simulink model "gm_detector"  (R2022a)
settings: Solver=FixedStepDiscrete  StartTime=0.0  StopTime=simTime  RelTol=1e-3
model workspace (MAT data in the model file):
  Sig = Simulink.Signal
  Sig.DataType = 'auto'
  Sig.Dimensions = -1
  Sig.DimensionsMode = 'auto'
  Sig.Complexity = 'auto'
  Sig.SampleTime = -1
  Sig.SamplingMode = 'auto'
libraries: dspsrcs4 x2
settings Model: Creator=ASAHIN  LastModifiedBy=alpha
settings SolverCC: AlgebraicLoopSolver=TrustRegion
settings OptimizationCC: BlockReduction=off  ConditionallyExecuteInputs=off  DefaultParameterBehavior=Inlined  InheritOutputTypeSmallerThanSingle=on
settings DebuggingCC: AlgebraicLoopMsg=error  InheritedTsInSrcMsg=none  SingleTaskRateTransMsg=error  UnconnectedInputMsg=warning  UnconnectedOutputMsg=warning  UnconnectedLineMsg=warning  SFMachineParentedDataDiag=warning
settings HardwareCC: ProdBitPerPointer=32  ProdBitPerSizeT=32  ProdBitPerPtrDiffT=32  ProdLargestAtomicFloat=None  ProdIntDivRoundTo=Undefined  ProdEndianess=Unspecified  ProdWordSize=32  ProdHWDeviceType=ASIC/FPGA->ASIC/FPGA  TargetBitPerPointer=64  TargetBitPerSizeT=64  TargetBitPerPtrDiffT=64  TargetLongLongMode=on  TargetIntDivRoundTo=Zero  TargetEndianess=LittleEndian  TargetWordSize=64  TargetHWDeviceType=Custom Processor->MATLAB Host Computer  ProdEqTarget=off
settings RTWCC: DLArmComputeVersion=19.05

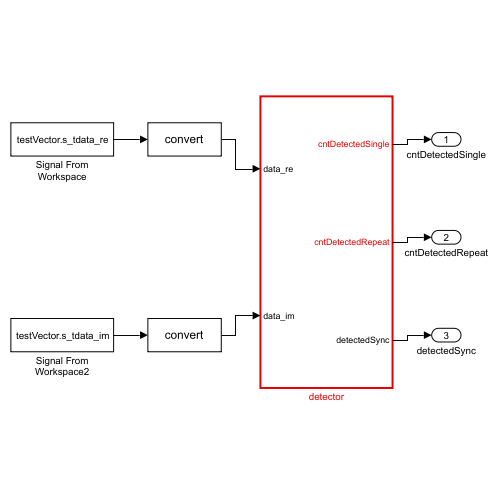
[thumbnail: Simulink's stored preview of the top-level diagram]
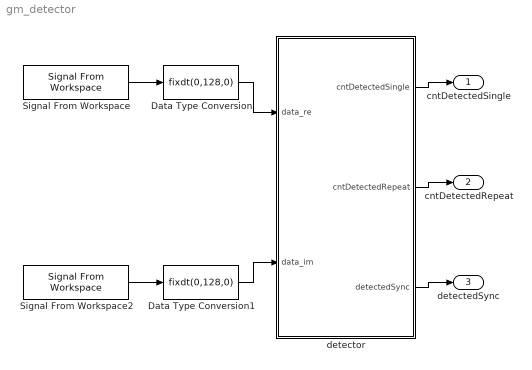
== system gm_detector ==
  Data Type Conversion : DataTypeConversion  OutDataTypeStr=fixdt(0,128,0)  SaturateOnIntegerOverflow=off  RndMeth=Floor
  Data Type Conversion1 : DataTypeConversion  OutDataTypeStr=fixdt(0,128,0)  SaturateOnIntegerOverflow=off  RndMeth=Floor
  Signal From Workspace : dspsrcs4/Signal From Workspace  X=testVector.s_tdata_re  Ts=1  nsamps=1  OutputAfterFinalValue=Setting to zero  ignoreOrWarnInputAndFrameLengths=off  OutputFrames=off
  Signal From Workspace2 : dspsrcs4/Signal From Workspace  X=testVector.s_tdata_im  Ts=1  nsamps=1  OutputAfterFinalValue=Setting to zero  ignoreOrWarnInputAndFrameLengths=off  OutputFrames=off
  detector : Subsystem  TreatAsAtomicUnit=on
  cntDetectedSingle : Outport
  cntDetectedRepeat : Outport  Port=2
  detectedSync : Outport  Port=3
  wires:
  Signal From Workspace/1 -> Data Type Conversion/1
  detector/1(cntDetectedSingle) -> cntDetectedSingle/1
  detector/3(detectedSync) -> detectedSync/1
  Data Type Conversion/1 -> detector/1(data_re)
  Signal From Workspace2/1 -> Data Type Conversion1/1
  detector/2(cntDetectedRepeat) -> cntDetectedRepeat/1
  Data Type Conversion1/1 -> detector/2(data_im)

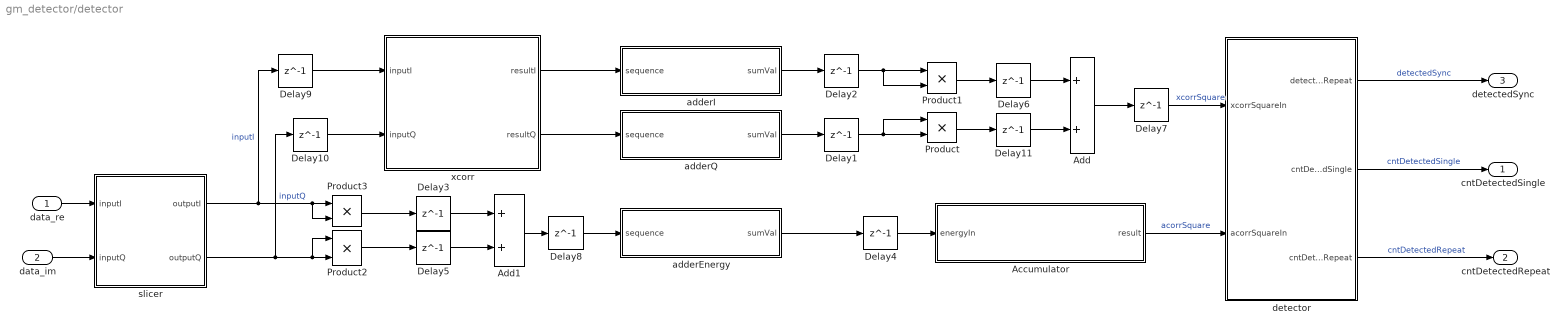
== system gm_detector/detector ==
  data_re : Inport
  data_im : Inport  Port=2
  Accumulator : MATLAB Function  TreatAsAtomicUnit=on
  Add : Sum
  Add1 : Sum
  Delay{1..11} (11 alike) : Delay  DelayLength=1  InitialCondition=0
  Product{,1..3} (4 alike) : Product
  adderEnergy : MATLAB Function  TreatAsAtomicUnit=on
  adderI : MATLAB Function  TreatAsAtomicUnit=on
  adderQ : MATLAB Function  TreatAsAtomicUnit=on
  detector : MATLAB Function  TreatAsAtomicUnit=on
  slicer : MATLAB Function  TreatAsAtomicUnit=on
  xcorr : MATLAB Function  TreatAsAtomicUnit=on
  cntDetectedSingle : Outport
  cntDetectedRepeat : Outport  Port=2
  detectedSync : Outport  Port=3
  wires:
  data_im/1 -> slicer/2(inputQ)
  data_re/1 -> slicer/1(inputI)
  Product/1 -> Delay11/1
  Delay11/1 -> Add/2
  Delay6/1 -> Add/1
  Delay5/1 -> Add1/2
  Delay3/1 -> Add1/1
  Delay2/1 -> Product1/1, Product1/2
  adderQ/1(sumVal) -> Delay1/1
  xcorr/2(resultQ) -> adderQ/1(sequence)
  xcorr/1(resultI) -> adderI/1(sequence)
  Add/1 -> Delay7/1
  detector/3(cntDetectedRepeat) -> cntDetectedRepeat/1  "cntDetectedRepeat"
  slicer/1(outputI) -> Delay9/1, Product3/1, Product3/2  "inputI"
  adderI/1(sumVal) -> Delay2/1
  slicer/2(outputQ) -> Delay10/1, Product2/2, Product2/1  "inputQ"
  Delay1/1 -> Product/1, Product/2
  detector/1(detectedRepeat) -> detectedSync/1  "detectedSync"
  Product2/1 -> Delay5/1
  Product3/1 -> Delay3/1
  Accumulator/1(result) -> detector/2(acorrSquareIn)  "acorrSquare"
  Delay10/1 -> xcorr/2(inputQ)
  Delay9/1 -> xcorr/1(inputI)
  Product1/1 -> Delay6/1
  Delay8/1 -> adderEnergy/1(sequence)
  Delay4/1 -> Accumulator/1(energyIn)
  Delay7/1 -> detector/1(xcorrSquareIn)  "xcorrSquare"
  adderEnergy/1(sumVal) -> Delay4/1
  detector/2(cntDetectedSingle) -> cntDetectedSingle/1  "cntDetectedSingle"
  Add1/1 -> Delay8/1

== matlab function gm_detector/detector/xcorr ==
  data: inputI input; resultI output; inputQ input; resultQ output; detectorSettings parameter
function [resultI, resultQ] = fcn_xcorr(inputI, inputQ, detectorSettings)
    inputI = inputI(:);
    inputQ = inputQ(:);
    Nsamples = size(inputI,1);
    sequenceBinary = ((detectorSettings.sequenceBPSK(:))+1)/2;
    sequenceBinary = fi(reshape(sequenceBinary,Nsamples,[]),0,1,0);
    Ntap = size(sequenceBinary,2);
    NbitEachXcorr = detectorSettings.NbitsSymbols+ceil(log2(Ntap));

    typeNbit = numerictype(1,NbitEachXcorr,0);

    %% Registers
    persistent delayIOutputs;
    if isempty(delayIOutputs)
        delayIOutputs = fi(zeros(Ntap,Nsamples),1,NbitEachXcorr,0);
    end    

    persistent delayQOutputs;
    if isempty(delayQOutputs)
        delayQOutputs = fi(zeros(Ntap,Nsamples),1,NbitEachXcorr,0);
    end        

    %% Set outputs
    resultI = delayIOutputs(end,:).';%sum(delayIOutputs(end,:));
    resultQ = delayQOutputs(end,:).';%sum(delayQOutputs(end,:));


    %% Update registers
    for indexXcorr = 1:Nsamples
        subSequence = sequenceBinary(indexXcorr,:);
        sumsResults = fi(zeros(Ntap-1,1),1,NbitEachXcorr,0);
        inputVal = inputI(indexXcorr);
        inputValNegated = -inputI(indexXcorr);
        if subSequence(1) == true
            inputP = inputVal;
        else
            inputP = inputValNegated;
        end
        for indSumResult = 1:Ntap-1
            if subSequence(indSumResult+1) == true
                sumsResults(indSumResult) = delayIOutputs(indSumResult,indexXcorr)+inputVal;
            else
                sumsResults(indSumResult) = delayIOutputs(indSumResult,indexXcorr)+inputValNegated;
            end
        end
        delayIOutputs(:,indexXcorr) = [fi(inputP,typeNbit); sumsResults];        
    end

    for indexXcorr = 1:Nsamples
        subSequence = sequenceBinary(indexXcorr,:);
        sumsResults = fi(zeros(Ntap-1,1),1,NbitEachXcorr,0);
        inputVal = inputQ(indexXcorr);
        inputValNegated = -inputQ(indexXcorr);
        if subSequence(1) == true
            inputP = inputVal;
        else
            inputP = inputValNegated;
        end
        for indSumResult = 1:Ntap-1
            if subSequence(indSumResult+1) == true
                sumsResults(indSumResult) = delayQOutputs(indSumResult,indexXcorr)+inputVal;
            else
                sumsResults(indSumResult) = delayQOutputs(indSumResult,indexXcorr)+inputValNegated;
            end
        end
        delayQOutputs(:,indexXcorr) = [fi(inputP,typeNbit); sumsResults];        
    end    
end

== matlab function gm_detector/detector/adderEnergy ==
  data: sequence input; sumVal output; detectorSettings parameter
function sumVal = fcn_adder(sequence, detectorSettings)
    NbitsOutput = 2*detectorSettings.NbitsSymbols+1 + ceil(log2(detectorSettings.Nsamples));



    %% Registers
    persistent sumVal_reg;
    if isempty(sumVal_reg)
        sumVal_reg = fi(0,1,NbitsOutput,0);
    end


    persistent level2;
    if isempty(level2)
        level2 = fi(zeros(1,2),1,NbitsOutput-1,0);
    end    
        

    persistent level1;
    if isempty(level1)
        level1 = fi(zeros(1,4),1,NbitsOutput-2,0);
    end

    
    %% Set outputs
    sumVal = sumVal_reg;

    %% Update registersa
    sumVal_reg = sum(fi(level2,1,NbitsOutput-1,0));    
    
    for i = 0:1
        level2(i+1) =  fi(level1(1+2*i),1,NbitsOutput-2,0) + fi(level1(2+2*i),1,NbitsOutput-2,0);
    end  

    for i = 0:3
        level1(i+1) = fi(sequence(1+2*i),1,NbitsOutput-3,0) + fi(sequence(2+2*i),1,NbitsOutput-3,0);
    end

== matlab function gm_detector/detector/detector ==
  settings: fimath=fimath('RoundingMethod', 'Floor','OverflowAction', 'Wrap','ProductMode', 'FullPrecision', 'SumMode', 'FullPrecision')
  data: xcorrSquareIn input; acorrSquareIn input; detectedRepeat output; cntDetectedSingle output; detectorSettings parameter; cntDetectedRepeat output
function [detectedRepeat,cntDetectedSingle, cntDetectedRepeat]  = fcn_comparator(xcorrSquareIn, acorrSquareIn, detectorSettings)
Lsequence = numel(detectorSettings.sequenceBPSK);
nbits = ceil(log2(Lsequence));
indices = Lsequence/detectorSettings.Nsamples*[0:detectorSettings.Nrepetitions-1]+1;

persistent detectionHistory;
if isempty(detectionHistory)
    detectionHistory = fi(zeros((detectorSettings.Nrepetitions-1)*Lsequence/detectorSettings.Nsamples+1,1),0,1,0);
end

persistent cntDetectedSingle_reg;
if isempty(cntDetectedSingle_reg)
    cntDetectedSingle_reg = uint16(0);
end 

persistent cntDetectedRepeat_reg;
if isempty(cntDetectedRepeat_reg)
    cntDetectedRepeat_reg = uint16(0);
end 

persistent detectedRepeat_reg;
if isempty(detectedRepeat_reg)
    detectedRepeat_reg = fi(0,0,1,0);
end 

persistent detectedSingle_reg;
if isempty(detectedSingle_reg)
    detectedSingle_reg = fi(0,0,1,0);
end 


detectedRepeat = detectedRepeat_reg;
cntDetectedSingle = cntDetectedSingle_reg;
cntDetectedRepeat = cntDetectedRepeat_reg;

detect = all(detectionHistory(indices) == fi(1,0,1,0)) == fi(1,0,1,0);
if detect == true
    cntDetectedRepeat_reg = cntDetectedRepeat_reg+1;
    detectedRepeat_reg = fi(1,0,1,0);
else
    detectedRepeat_reg = fi(0,0,1,0);
end


if  detectedSingle_reg == fi(1,0,1,0)
    detectionHistory = [fi(1,0,1,0); detectionHistory(1:end-1)];
    cntDetectedSingle_reg = cntDetectedSingle_reg+1;
else
    detectionHistory = [fi(0,0,1,0); detectionHistory(1:end-1)];
end


if  bitsra(xcorrSquareIn,nbits-2) >  acorrSquareIn
    detectedSingle_reg = fi(1,0,1,0);
else
    detectedSingle_reg = fi(0,0,1,0);
end

== matlab function gm_detector/detector/Accumulator ==
  settings: fimath=fimath('RoundingMethod', 'Floor','OverflowAction', 'Wrap','ProductMode', 'FullPrecision', 'SumMode', 'FullPrecision')
  data: energyIn input; result output; detectorSettings parameter
function result = fcn_accumulator(energyIn, detectorSettings)
    Ntaps = numel(detectorSettings.sequenceBPSK)/detectorSettings.Nsamples;
    NbitsEnergy = 2*detectorSettings.NbitsSymbols+1+log2(detectorSettings.Nsamples);
    numberOfBitsEnergy = NbitsEnergy+ceil(log2(Ntaps));
    
    %% Registers
    persistent delayOutputs;
    if isempty(delayOutputs)
        delayOutputs = fi(zeros(Ntaps,1),1,NbitsEnergy,0);
    end
    persistent energy;
    if isempty(energy)
        energy = fi(0,1,numberOfBitsEnergy,0);
    end

    persistent diffEnergy;
    if isempty(diffEnergy)
        diffEnergy = fi(0,1,numberOfBitsEnergy-1,0);
    end    

    %energyIn = fi(energyIn,0,numberOfBitsDelay,0,'RoundingMethod','floor', 'SumMode','FullPrecision','ProductMode','FullPrecision'); 

    %% Set outputs
    result = energy; 
    
    %% Update registers
    energyOut = delayOutputs(end);
    delayOutputs(2:end) = delayOutputs(1:end-1);
    delayOutputs(1) = energyIn;
    %aa = fi(energy,1,numberOfBitsEnergy-2,0) + fi(energyIn,1,numberOfBitsEnergy-2,0) - fi(energyOut,1,numberOfBitsEnergy-2,0); % Full implementation
    %energy = aa;

    energy = fi(energy,1,numberOfBitsEnergy-1,0)  + diffEnergy;
    diffEnergy = fi(energyIn,1,numberOfBitsEnergy-2,0) - fi(energyOut,1,numberOfBitsEnergy-2,0);
end

== matlab function gm_detector/detector/slicer ==
  settings: fimath=fimath('RoundingMethod', 'Floor','OverflowAction', 'Wrap','ProductMode', 'FullPrecision', 'SumMode', 'FullPrecision')
  data: inputI input; inputQ input; outputI output; outputQ output; detectorSettings parameter
function [outputI, outputQ]= fcn_slicer(inputI, inputQ, detectorSettings)

outputIu = fi(zeros(8,1),0,detectorSettings.NbitsSymbols,0);
outputQu = fi(zeros(8,1),0,detectorSettings.NbitsSymbols,0);

sampleIndex = 1;
outputIu(sampleIndex) = bitsliceget(inputI,sampleIndex*16-(16-detectorSettings.NbitsSymbols),(sampleIndex-1)*16+1);
outputQu(sampleIndex) = bitsliceget(inputQ,sampleIndex*16-(16-detectorSettings.NbitsSymbols),(sampleIndex-1)*16+1);

sampleIndex = 2;
outputIu(sampleIndex) = bitsliceget(inputI,sampleIndex*16-(16-detectorSettings.NbitsSymbols),(sampleIndex-1)*16+1);
outputQu(sampleIndex) = bitsliceget(inputQ,sampleIndex*16-(16-detectorSettings.NbitsSymbols),(sampleIndex-1)*16+1);

sampleIndex = 3;
outputIu(sampleIndex) = bitsliceget(inputI,sampleIndex*16-(16-detectorSettings.NbitsSymbols),(sampleIndex-1)*16+1);
outputQu(sampleIndex) = bitsliceget(inputQ,sampleIndex*16-(16-detectorSettings.NbitsSymbols),(sampleIndex-1)*16+1);

sampleIndex = 4;
outputIu(sampleIndex) = bitsliceget(inputI,sampleIndex*16-(16-detectorSettings.NbitsSymbols),(sampleIndex-1)*16+1);
outputQu(sampleIndex) = bitsliceget(inputQ,sampleIndex*16-(16-detectorSettings.NbitsSymbols),(sampleIndex-1)*16+1);

sampleIndex = 5;
outputIu(sampleIndex) = bitsliceget(inputI,sampleIndex*16-(16-detectorSettings.NbitsSymbols),(sampleIndex-1)*16+1);
outputQu(sampleIndex) = bitsliceget(inputQ,sampleIndex*16-(16-detectorSettings.NbitsSymbols),(sampleIndex-1)*16+1);

sampleIndex = 6;
outputIu(sampleIndex) = bitsliceget(inputI,sampleIndex*16-(16-detectorSettings.NbitsSymbols),(sampleIndex-1)*16+1);
outputQu(sampleIndex) = bitsliceget(inputQ,sampleIndex*16-(16-detectorSettings.NbitsSymbols),(sampleIndex-1)*16+1);

sampleIndex = 7;
outputIu(sampleIndex) = bitsliceget(inputI,sampleIndex*16-(16-detectorSettings.NbitsSymbols),(sampleIndex-1)*16+1);
outputQu(sampleIndex) = bitsliceget(inputQ,sampleIndex*16-(16-detectorSettings.NbitsSymbols),(sampleIndex-1)*16+1);

sampleIndex = 8;
outputIu(sampleIndex) = bitsliceget(inputI,sampleIndex*16-(16-detectorSettings.NbitsSymbols),(sampleIndex-1)*16+1);
outputQu(sampleIndex) = bitsliceget(inputQ,sampleIndex*16-(16-detectorSettings.NbitsSymbols),(sampleIndex-1)*16+1);

T16 = numerictype(1,detectorSettings.NbitsSymbols,0);
outputI = fi(outputIu,T16);
outputQ = fi(outputQu,T16);

end

== matlab function gm_detector/detector/adderI ==
  data: sequence input; sumVal output; detectorSettings parameter
function sumVal = fcn_adder(sequence, detectorSettings)

    NbitsOutput = detectorSettings.NbitsSymbols +ceil(log2(numel(detectorSettings.sequenceBPSK)));
    
    %% Registers
    persistent sumVal_reg;
    if isempty(sumVal_reg)
        sumVal_reg = fi(0,1,NbitsOutput,0);
    end
    
    
    persistent level2;
    if isempty(level2)
        level2 = fi(zeros(1,2),1,NbitsOutput-1,0);
    end
    
    
    persistent level1;
    if isempty(level1)
        level1 = fi(zeros(1,4),1,NbitsOutput-2,0);
    end
    
    
    %% Set outputs
    sumVal = sumVal_reg;
    
    %% Update registersa
    sumVal_reg = sum(fi(level2,1,NbitsOutput-1,0));
    
    for ind = 0:1
        level2(ind+1) =  fi(level1(1+2*ind),1,NbitsOutput-2,0) + fi(level1(2+2*ind),1,NbitsOutput-2,0);
    end
    
    for ind = 0:3
        level1(ind+1) = fi(sequence(1+2*ind),1,NbitsOutput-3,0) + fi(sequence(2+2*ind),1,NbitsOutput-3,0);
    end

== matlab function gm_detector/detector/adderQ ==
  data: sequence input; sumVal output; detectorSettings parameter
function sumVal = fcn_adder(sequence, detectorSettings)
    NbitsOutput = detectorSettings.NbitsSymbols +ceil(log2(numel(detectorSettings.sequenceBPSK)));
    
    %% Registers
    persistent sumVal_reg;
    if isempty(sumVal_reg)
        sumVal_reg = fi(0,1,NbitsOutput,0);
    end


    persistent level2;
    if isempty(level2)
        level2 = fi(zeros(1,2),1,NbitsOutput-1,0);
    end    
        

    persistent level1;
    if isempty(level1)
        level1 = fi(zeros(1,4),1,NbitsOutput-2,0);
    end

    
    %% Set outputs
    sumVal = sumVal_reg;

    %% Update registersa
    sumVal_reg = sum(fi(level2,1,NbitsOutput-1,0));    
    
    for ind = 0:1
        level2(ind+1) =  fi(level1(1+2*ind),1,NbitsOutput-2,0) + fi(level1(2+2*ind),1,NbitsOutput-2,0);
    end  

    for ind = 0:3
        level1(ind+1) = fi(sequence(1+2*ind),1,NbitsOutput-3,0) + fi(sequence(2+2*ind),1,NbitsOutput-3,0);
    end
